simulink model "charge_controller"  (R2026a)
settings: Solver=FixedStepAuto
values from neighbouring files (symbols this model uses):
  Ts = 1.0E-6    [vars.sldd]
libraries: slpidlib x1, eePwmGenerator x1, simulink x1
settings Model: DataDictionary=vars.sldd  Creator=caden  LastModifiedBy=cra0035

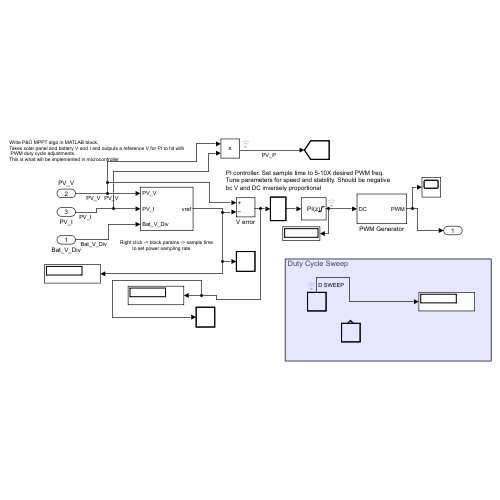
[thumbnail: Simulink's stored preview of the top-level diagram]
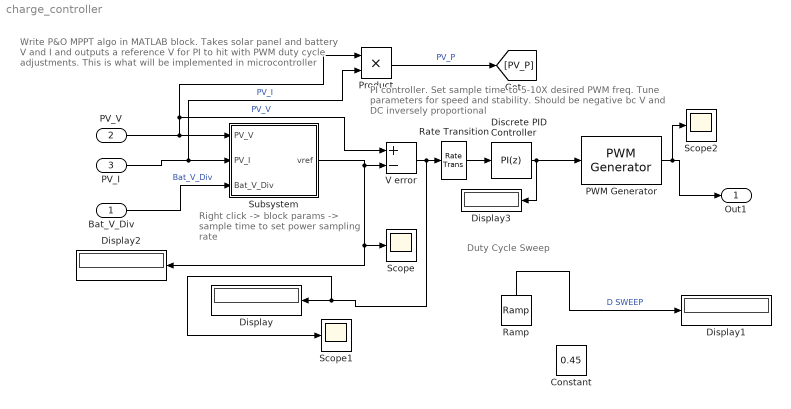
== system charge_controller ==
  note: Duty Cycle Sweep
  note: PI controller. Set sample time to 5-10X desired PWM freq.
      | Tune parameters for speed and stability. Should be negative
      | bc V and DC inversely proportional
  note: Right click -> block params -> sample time
      | to set power sampling rate
  note: Write P&O MPPT algo in MATLAB block.
      | Takes solar panel and battery V and I and outputs a reference V for PI to hit with
      | PWM duty cycle adjustments.
      | This is what will be implemented in microcontroller
  Bat_V_Div : Inport
  PV_V : Inport  Port=2  SampleTime=Ts
  PV_I : Inport  Port=3  SampleTime=Ts
  Constant : Constant  Value=0.45
  Discrete PID Controller : slpidlib/PID Controller  Controller=PI  Form=Parallel  TimeDomain=Discrete-time  UseExternalTs=off  SampleTime=1e-4  IntegratorMethod=Backward Euler  FilterMethod=Forward Euler  ControllerParametersSource=internal  P=0.0015  I=0.00025  UseKiTs=on  D=0  UseExternalDerivativeSource=off  N=100  UseFilter=on  TunerSelectOption=Transfer Function Based (PID Tuner App)  InitialConditionSource=internal  InitialConditionForIntegrator=0.5  InitialConditionForFilter=0  DifferentiatorICPrevScaledInput=0  ExternalReset=none  TrackingMode=off  Kt=1  LimitOutput=on  SatLimitsSource=internal  UpperSaturationLimit=0.95  LowerSaturationLimit=0.05  LinearizeAsGain=off  AntiWindupMode=none  Kb=1  LimitIntegrator=on  UpperIntegratorSaturationLimit=0.95  LowerIntegratorSaturationLimit=0.05  POutMin=[]  POutMax=[]  IOutMin=[]  IOutMax=[]  DOutMin=[]  DOutMax=[]  NOutMin=[]  NOutMax=[]  SumOutMin=[]  SumOutMax=[]  SaturationOutMin=[]  SaturationOutMax=[]  PParamMin=[]  PParamMax=[]  IParamMin=[]  IParamMax=[]  DParamMin=[]  DParamMax=[]  NParamMin=[]  NParamMax=[]  KbParamMin=[]  KbParamMax=[]  KtParamMin=[]  KtParamMax=[]  KbOutMin=[]  KbOutMax=[]  KtOutMin=[]  KtOutMax=[]  IntegratorOutMin=[]  IntegratorOutMax=[]  FilterOutMin=[]  FilterOutMax=[]  SumI1OutMin=[]  SumI1OutMax=[]  SumI2OutMin=[]  SumI2OutMax=[]  SumI3OutMin=[]  SumI3OutMax=[]  SumI4OutMin=[]  SumI4OutMax=[]  SumDOutMin=[]  SumDOutMax=[]  DifferentiatorOutMin=[]  DifferentiatorOutMax=[]  FilterDiffOutCoefMin=[]  FilterDiffOutCoefMax=[]  ReciprocalOutMin=[]  ReciprocalOutMax=[]  SumDenOutMin=[]  SumDenOutMax=[]  SumNumOutMin=[]  SumNumOutMax=[]  DivideOutMin=[]  DivideOutMax=[]  UdiffTsProdOutMin=[]  UdiffTsProdOutMax=[]  NTsProdOutMin=[]  NTsProdOutMax=[]  UintegralTsProdOutMin=[]  UintegralTsProdOutMax=[]  UngainTsProdOutMin=[]  UngainTsProdOutMax=[]  ClampingZeroOutDataTypeStr=Inherit: Inherit via back propagation  ClampingZeroOutMin=[]  ClampingZeroOutMax=[]  FilterDenConstantOutDataTypeStr=Inherit: Inherit via back propagation  FilterDenConstantOutMin=[]  FilterDenConstantOutMax=[]  PCopyOutDataTypeStr=Inherit: Inherit via back propagation  PCopyOutMin=[]  PCopyOutMax=[]  NCopyOutDataTypeStr=Inherit: Inherit via back propagation  NCopyOutMin=[]  NCopyOutMax=[]  IntegratorContinuousStateAttributes=''  IntegratorStateMustResolveToSignalObject=off  IntegratorRTWStateStorageClass=Auto  FilterContinuousStateAttributes=''  FilterStateMustResolveToSignalObject=off  FilterRTWStateStorageClass=Auto  ParallelPVariant=InternalParameters  IdealPVariant=Disabled  IVariant=InternalParameters  DVariant=Disabled  IntegratorVariant=Discrete  SatVariant=Enabled  AWVariant=Passthrough  PCopyVariant=Disabled  TRVariant=Disabled  FdbkBlocksVariant=Forward  IdealPFdbkVariant=Disabled  SatFdbkVariant=Disabled  DerivativeFilterVariant=Disabled  NVariant=Disabled  NCopyVariant=Disabled_SignalSpec  FilterICVariant=Disabled  IntegratorICVariant=InternalICs  ExternalResetVariant=Disabled  TRSumVariant=Passthrough  SumFdbkVariant=Disabled  SumVariant=Sum_PI  TsampFilterVariant=InternalTs  TsampNgainVariant=Passthrough  TsampIntegralVariant=Disabled_SignalSpec  ExternalSaturationOutDataTypeStr=Inherit: Same as second input  DerivativeSourceVariant=Disabled  PreIntVariant=InternalPreInt
      settings: LibrarySourceBlock=simulink/Discrete/Discrete PID Controller
  Display{,1..3} (4 alike) : Display
  PWM Generator : eePwmGenerator/PWM Generator  CarrCount=Up  Tper=1e-5  Tdelay=0  Ts=Ts
  Product : Product
  Ramp : simulink/Sources/Ramp  slope=0.09  start=0  InitialOutput=0.05
  Rate Transition : RateTransition
  Scope : Scope
      settings: ActiveDisplayYMinimum=6.2747153613209665  ActiveDisplayYMaximum=22.3659342969565
  Scope1 : Scope
      settings: ActiveDisplayYMinimum=-1  ActiveDisplayYMaximum=1
  Scope2 : Scope
      settings: ActiveDisplayYMinimum=0.0085180998474295166  ActiveDisplayYMaximum=0.93092251103500723  DataLoggingVariableName=ScopeData2
  Subsystem : Subsystem
  V error : Sum  Inputs=+-
  Out1 : Outport
  wires:
  PWM Generator/1 -> Out1/1, Scope2/1
  Rate Transition/1 -> Discrete PID Controller/1
  V error/1 -> Scope1/1, Display/1, Rate Transition/1
  Product/1 -> [PV_P]  "PV_P"
  Subsystem/1(vref) -> Display2/1, Scope/1, V error/2
  PV_V/1 -> Subsystem/1(PV_V), V error/1, Product/1  "PV_V"
  Bat_V_Div/1 -> Subsystem/3(Bat_V_Div)  "Bat_V_Div"
  PV_I/1 -> Subsystem/2(PV_I), Product/2  "PV_I"
  Ramp/1 -> Display1/1  "D SWEEP"
  Discrete PID Controller/1 -> PWM Generator/1, Display3/1

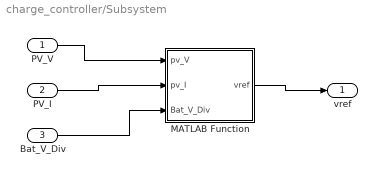
== system charge_controller/Subsystem ==
  PV_V : Inport
  PV_I : Inport  Port=2
  Bat_V_Div : Inport  Port=3
  MATLAB Function : MATLAB Function  TreatAsAtomicUnit=on  SystemSampleTime=0.01
  vref : Outport
  wires:
  MATLAB Function/1(vref) -> vref/1
  PV_V/1 -> MATLAB Function/1(pv_V)
  Bat_V_Div/1 -> MATLAB Function/3(Bat_V_Div)
  PV_I/1 -> MATLAB Function/2(pv_I)

== matlab function charge_controller/Subsystem/MATLAB Function ==
  data: pv_V input; vref output; pv_I input; Bat_V_Div input
% 3 charge states: 
% 1. Bulk (mppt): battery low or mid. Route max power
% 2. Absorption: battery nearly full, stop MPPT and hold V at high level
% 3. Float: Battery 100% charged. Sit at slightly lower V to maintain
% charge w/o overcharging
function vref = ChargeController(pv_V,pv_I,Bat_V_Div)
    persistent charge_state P_old V_mpp_tracked;
    V_DIV_RATIO = 5; %Set to (Big R + Small R)/Small R of bat V divider
    bat_V = Bat_V_Div * V_DIV_RATIO; %This should recover the bat's actual V
    V_STEP = 0.05; % Tune me!
    V_MAX = 48;%21.8; %Voc
    V_MIN = 12.0;
    V_ABSORPTION = 14.4; %battery voltage when full
    V_FLOAT = 13.5; %Maintenance V, prevent overcharge
    V_INITIAL_GUESS = 31.9; %Best to guess operating voltage initially


   
   
   
   % INITIAL (BOOT)
   if isempty(charge_state)
        charge_state = 1; %bulk
        V_mpp_tracked = V_INITIAL_GUESS; %Guess the initial voltage to track (rated V)
        P_old = 0;
   end
   pv_P = pv_V * pv_I; %Current panel power

   %CHARGING STATE MACHINE
   if charge_state == 1 % 1. BULK
        if bat_V >= V_ABSORPTION %Close to full?
            charge_state = 2; %enter absorption state
            vref = V_mpp_tracked;
        else %do P&O
            vref = Piano(pv_V, pv_P, V_mpp_tracked, P_old, V_STEP, V_MAX, V_MIN);
            V_mpp_tracked = vref;
            P_old = pv_P;
        end

   elseif charge_state == 2 % 2. ABSORPTION (80-85% full)
        if bat_V >= (V_ABSORPTION + 0.1) % Battery V too high
            vref = V_mpp_tracked + V_STEP; % Increase pv voltage
        elseif bat_V < V_ABSORPTION       % Battery V too low
            vref = V_mpp_tracked - V_STEP;  % Decrease pv voltage
        else     % Battery V good
            vref = V_mpp_tracked;
        end

   else % 3. FLOAT (~100% full)
       if bat_V >= (V_FLOAT + 0.1) % Battery V too high
           vref = V_mpp_tracked + V_STEP; % Increase pv voltage
       elseif bat_V < V_FLOAT       % Battery V too low
           vref = V_mpp_tracked - V_STEP;  % Decrease pv voltage
       else     % Battery V good
           vref = V_mpp_tracked;
       end
        % I don't know how to implement transition to/from float yet.
        % Can use timer (~1hr) or track battery current to decide when full
   end
   
end

%---MPPT----
% Perturb & Observe (P&O)
function vref_out = Piano(pv_V, pv_P, V_old, P_old, v_step, v_max, v_min)
    
    dP = pv_P-P_old;
    dV = pv_V-V_old;
    if dP > 0
        if dV > 0
            vref_out = V_old + v_step;
        else
            vref_out = V_old - v_step;
        end
    else
        if dV > 0
            vref_out = V_old - v_step;
        else
            vref_out = V_old + v_step;
        end
    end

    % Boundaries
    vref_out = max(v_min, min(v_max,vref_out));
end
